simulink model "lab1_closedLoop_sim"  (R2020b)
settings: Solver=VariableStepAuto  StartTime=0.0  StopTime=10.0  RelTol=1e-3
settings Model: Creator=MSI  LastModifiedBy=berksahin

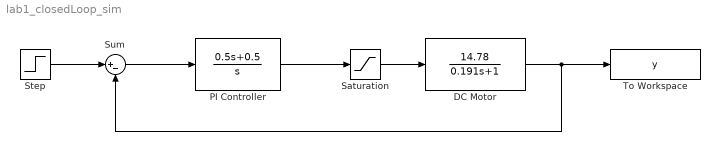
== system lab1_closedLoop_sim ==
  DC Motor : TransferFcn  Numerator=[14.78]  Denominator=[0.191 1]
  PI Controller : TransferFcn  Numerator=[0.5 0.5]  Denominator=[1 0]
  Saturation : Saturate  UpperLimit=12  LowerLimit=-12
  Step : Step  Time=0  After=20  SampleTime=0
  Sum : Sum  Inputs=|+-
  To Workspace : ToWorkspace  VariableName=y  SaveFormat=Timeseries  SampleTime=-1
  wires:
  PI Controller/1 -> Saturation/1
  Saturation/1 -> DC Motor/1
  DC Motor/1 -> Sum/2, To Workspace/1
  Sum/1 -> PI Controller/1
  Step/1 -> Sum/1
